simulink library "simeventsuserdefined1"  (Simulink 7.0)
undefined symbols (not defined in the file or in its folder): des_attributefunction_support
libraries: simeventsattributes2 x2, simeventstranslate1 x1
settings Model: Creator=aapte  LastModifiedBy=Liw  ExtModeAutoUpdateStatusClock=off

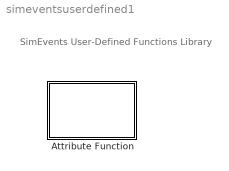
== system simeventsuserdefined1 ==
  note: SimEvents User-Defined Functions Library
  Attribute Function : Subsystem  LoadFcn=des_attributefunction_support(gcb,'LoadFcn');  StartFcn=des_attributefunction_support(gcb,'StartFcn');  mask(Attribute Function){OutputNamePrefix=out_}
      mask prompts: OutputNamePrefix "Prefix name"
      settings: CopyFcn=des_attributefunction_support(gcb,'CopyFcn');  OpenFcn=des_attributefunction_support(gcb,'OpenFcn');  ErrorFcn=des_error_redirect
      mask Help: helpview(simeventsbhelp('attributefunction'))
      mask Display: image(des_iconLoad('attribFunction.jpg'),'center');

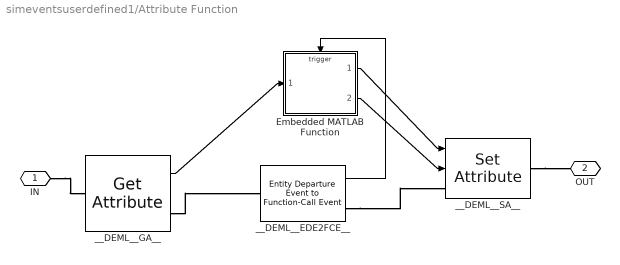
== system simeventsuserdefined1/Attribute Function ==
  Embedded MATLAB Function : Stateflow chart
      settings: PropExecContextOutsideSubsystem=on
  __DEML__EDE2FCE__ : simeventstranslate1/Entity Departure Event to Function-Call Event  Priority=1  SystemSampleTime=-1  TimingFunctionCallF1=Before entity departure  EnableE1Port=off  EnableF2Port=off  TimingFunctionCallF2=Before entity departure  EnableE2Port=off  StatNumberDeparted=Off  StatNumberF1Calls=Off  StatNumberF2Calls=Off  IsInsideAFB=on
  __DEML__GA__ : simeventsattributes2/Get Attribute  Priority=1  DialogController=des_ddg_create  DialogControllerArgs=DataTag2  SystemSampleTime=-1  AttributeName=Attribute1  AttributeMissing=Error  AttributeDefaultValue=1  AttributeSendTiming=Before entity departure  AttributeTreatAsVector=1  StatNumberDeparted=Off  EvaluatedDefaultAttributeValue=0
  __DEML__SA__ : simeventsattributes2/Set Attribute  Priority=1  DialogController=des_ddg_create  DialogControllerArgs=DataTag4  SystemSampleTime=-1  AttributeFrom=Signal port|Signal port  AttributeName=Attribute1|Attribute2  AttributeTreatAsVector=1|1  AttributeValue=1|1  AttributeCreate=on  StatNumberDeparted=Off  EvaluatedAttributeValue=0
  IN : PMIOPort  Port=1  Side=Left
  OUT : PMIOPort  Orientation=left  Port=2  Side=Right
  wires:
  __DEML__EDE2FCE__/1 -> Embedded MATLAB Function/Trigger
  __DEML__GA__/1 -> Embedded MATLAB Function/1(Attribute1)
  Embedded MATLAB Function/1(out_Attribute1) -> __DEML__SA__/1
  Embedded MATLAB Function/2(out_Attribute2) -> __DEML__SA__/2
  connections:
  __DEML__EDE2FCE__/RConn1 -- __DEML__SA__/LConn1
  __DEML__GA__/RConn1 -- __DEML__EDE2FCE__/LConn1
  IN/RConn1 -- __DEML__GA__/LConn1
  __DEML__SA__/RConn1 -- OUT/RConn1

== matlab function Attribute Function/Embedded MATLAB Function ==
  data: Attribute1 input inherited; out_Attribute1 output inherited; out_Attribute2 output inherited
  events: trigger input FUNCTION_CALL_EVENT
function [out_Attribute1, out_Attribute2] = fcn(Attribute1)
%FCN    Access and modify attributes with Embedded MATLAB Function 
% 
% Input arguments must match the attribute names.
% Output arguments must be out_<AttributeName>,
% e.g., out_ServiceTime where ServiceTime is the attribute name.
% 
% The output attribute will be created if it is not present.
%

out_Attribute1 = Attribute1 + 1;
out_Attribute2 = Attribute1*2;
